simulink model "P4_sim"  (R2012b)
settings: Solver=ode45  StartTime=0.0  StopTime=tsim  RelTol=1e-3
values from neighbouring files (symbols this model uses):
  A = [0, 1, 0; 0, 0, 1; -1, -2, -3]    [P4.m]
  Am = A + B * K    [P4.m]
  B = [0, 0; 1, 0; -1, 2]    [P4.m]    (also in p1d.m = [-1, -3; 0, -1])
  Bp = B * Lambda    [P4.m]
  CRMs = 1    [P4.m]
  Gamma_p = 10 * eye(m)    [P4.m]
  Gamma_t = 10 * eye(m)    [P4.m]
  L = L'    [P4.m]
  P = lyap(Aml', Q')    [P4.m]
  phi_0 = zeros(m,m)    [P4.m]
  theta_0 = zeros(m,n)    [P4.m]
  x0 = 2*ones(n,1)    [P4.m]
  xm0 = 0*ones(n,1)    [P4.m]
settings Model: Creator=Zheng Qu  LastModifiedBy=mzqu

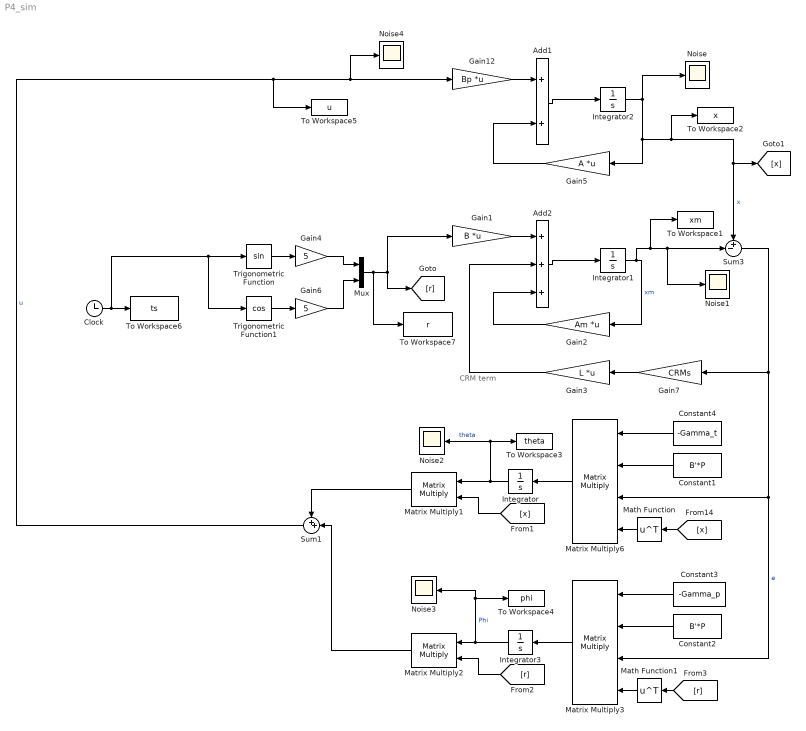
== system P4_sim ==
  note: CRM term
  Add1 : Sum  Inputs=2
  Add2 : Sum  Inputs=3
  Clock : Clock
  Constant1 : Constant  Value=B'*P  VectorParams1D=off
  Constant2 : Constant  Value=B'*P  VectorParams1D=off
  Constant3 : Constant  Value=-Gamma_p  VectorParams1D=off
  Constant4 : Constant  Value=-Gamma_t  VectorParams1D=off
  Gain1 : Gain  Gain=B  Multiplication=Matrix(K*u)
  Gain12 : Gain  Gain=Bp  Multiplication=Matrix(K*u)
  Gain2 : Gain  Gain=Am  Multiplication=Matrix(K*u)
  Gain3 : Gain  Gain=L  Multiplication=Matrix(K*u)
  Gain4 : Gain  Gain=5
  Gain5 : Gain  Gain=A  Multiplication=Matrix(K*u)
  Gain6 : Gain  Gain=5
  Gain7 : Gain  Gain=CRMs
  Integrator : Integrator  InitialCondition=theta_0
  Integrator1 : Integrator  InitialCondition=xm0
  Integrator2 : Integrator  InitialCondition=x0
  Integrator3 : Integrator  InitialCondition=phi_0
  Math Function : Math  Operator=transpose  SaturateOnIntegerOverflow=on
  Math Function1 : Math  Operator=transpose  SaturateOnIntegerOverflow=on
  Matrix Multiply1 : Product  Multiplication=Matrix(*)
  Matrix Multiply2 : Product  Multiplication=Matrix(*)
  Matrix Multiply3 : Product  Inputs=4  Multiplication=Matrix(*)
  Matrix Multiply6 : Product  Inputs=4  Multiplication=Matrix(*)
  Mux : Mux  Inputs=2
  Noise{,1..4} (5 alike) : Scope
      Noise settings: ShowLegends=on  TimeRange=20  SaveName=Theta  Decimation=data_deci
      Noise1 settings: ShowLegends=on  TimeRange=20  SaveName=Theta1  Decimation=data_deci
      Noise2 settings: ShowLegends=on  TimeRange=20  SaveName=Theta2  Decimation=data_deci
      Noise3 settings: ShowLegends=on  TimeRange=20  SaveName=Theta3  Decimation=data_deci
      Noise4 settings: ShowLegends=on  TimeRange=20  SaveName=Theta4  Decimation=data_deci
  Sum1 : Sum  Inputs=++|
  Sum3 : Sum  Inputs=+-|
  To Workspace1 : ToWorkspace  VariableName=xm  SampleTime=-1
      settings: Decimation=data_deci
  To Workspace2 : ToWorkspace  VariableName=x  SampleTime=-1
      settings: Decimation=data_deci
  To Workspace3 : ToWorkspace  VariableName=theta  SampleTime=-1
      settings: Decimation=data_deci
  To Workspace4 : ToWorkspace  VariableName=phi  SampleTime=-1
      settings: Decimation=data_deci
  To Workspace5 : ToWorkspace  VariableName=u  SampleTime=-1
      settings: Decimation=data_deci
  To Workspace6 : ToWorkspace  VariableName=ts  SampleTime=-1
      settings: Decimation=data_deci
  To Workspace7 : ToWorkspace  VariableName=r  SampleTime=-1
      settings: Decimation=data_deci
  Trigonometric Function : Trigonometry
  Trigonometric Function1 : Trigonometry  Operator=cos
  wires:
  Add1/1 -> Integrator2/1
  Integrator2/1 -> Noise/1, [x], Sum3/1, To Workspace2/1, Gain5/1  "x"
  Gain5/1 -> Add1/2
  Add2/1 -> Integrator1/1
  Integrator1/1 -> Gain2/1, To Workspace1/1, Noise1/1, Sum3/2  "xm"
  Gain2/1 -> Add2/3
  Gain1/1 -> Add2/1
  Sum3/1 -> Matrix Multiply3/3, Matrix Multiply6/3, Gain7/1  "e"
  Gain3/1 -> Add2/2
  Constant4/1 -> Matrix Multiply6/1
  Constant1/1 -> Matrix Multiply6/2
  [x] -> Math Function/1
  Matrix Multiply6/1 -> Integrator/1
  Integrator/1 -> Matrix Multiply1/1, Noise2/1, To Workspace3/1  "theta"
  [x] -> Matrix Multiply1/2
  Matrix Multiply1/1 -> Sum1/1
  Constant3/1 -> Matrix Multiply3/1
  Constant2/1 -> Matrix Multiply3/2
  [r] -> Math Function1/1
  Matrix Multiply3/1 -> Integrator3/1
  Integrator3/1 -> Noise3/1, To Workspace4/1, Matrix Multiply2/1  "Phi"
  [r] -> Matrix Multiply2/2
  Matrix Multiply2/1 -> Sum1/2
  Math Function/1 -> Matrix Multiply6/4
  Math Function1/1 -> Matrix Multiply3/4
  Sum1/1 -> To Workspace5/1, Noise4/1, Gain12/1  "u"
  Gain12/1 -> Add1/1
  Clock/1 -> Trigonometric Function1/1, Trigonometric Function/1, To Workspace6/1
  Trigonometric Function/1 -> Gain4/1
  Trigonometric Function1/1 -> Gain6/1
  Gain4/1 -> Mux/1
  Gain6/1 -> Mux/2
  Mux/1 -> To Workspace7/1, [r], Gain1/1
  Gain7/1 -> Gain3/1
